simulink model "main_RI_LIEKF"  (R2023a)
settings: Solver=FixedStepAuto  StartTime=0.0  StopTime=220  FixedStep=0.01  RelTol=1e-3
InitFcn:
  | initNavigation0612_AOA;
values from neighbouring files (symbols this model uses):
  CF_enable = 0    [initNavigation.m]
  dt = 0.01    [initNavigation.m]
  dtDelay = -0.03    [initNavigation.m]
  g0 = 9.795    [initNavigation.m]
  gam0_rad = 0/57.3    (= 0)    [initNavigation.m]
  H_sensor_type = 0    [initNavigation.m]
  KF_enable = 1    [initNavigation.m]
  P0 = diag([1*ones(3,1);0.01*ones(3,1);0.1*ones(3,1);0.001*ones(3,1);0.00001*ones(3,1)])    [initNavigation.m]
  P0_RIEKF = diag([1*ones(3,1);0.01*ones(3,1);0.1*ones(3,1);0.001*ones(3,1);0.00001*ones(3,1);      0.01*ones(3,1);[0;2;2]/57.3;[0.1;0.1;0.1]])^2    [initNavigation.m]
  pd0 = 0    [initNavigation.m]
  pe0 = 0    [initNavigation.m]
  phi0_rad = 0/57.3    (= 0)    [initNavigation.m]
  pn0 = 0    [initNavigation.m]
  psi = -178    [initNavigation.m]
  psi0_rad = 0/57.3    (= 0)    [initNavigation.m]
  state_dim = 24    [initNavigation.m]
  Time = 0:0.01:(size(traindata.AttackAngle,1) - 1)*0.01    [NNLiftCoefficientFit.m]
  vd0 = 0    [initNavigation.m]
  ve0 = 0    [initNavigation.m]
  vn0 = 0    [initNavigation.m]
undefined symbols (not defined in the file or in its folder): DiscIntNeverNeededParam, Discrete, INS_CONST, INS_EXPORT, INS_PARAM, magnitude, p, param, pInitialization, sys
libraries: simulink x69, simulink_extras x64, dspstat3 x56, sharedtransform x49, ctrlSharedLib x36, sharedTrackingLibrary x17, FMT_Model_Lib x13, matrix_library x12, deeplib x4, dspsolvers x4, vrlib x4, aerolibconvert2 x1
(part 2 of 22)

== system main_RI_LIEKF/Sensor_Data_Process/Magn_Data_Process1/Mag_Data_Process ==
  mag_B_uT : Inport
  mag_valid : Inport  Port=2
  DCM_OB : Inport  Port=3
  GPS_Data : Inport  Port=4
  Bus Selector : BusSelector  OutputSignals=lat_gps,lon_gps
  Bus Selector1 : BusSelector  OutputSignals=fixtype_gps
  Compare To Constant : simulink/Logic and Bit Operations/Compare To Constant  relop=>=  const=1  OutDataTypeStr=boolean
  Mag_Quality_Estimate : Subsystem
  Scope : Scope
  WMM_Compensation : Subsystem
  WMM_LUT : Subsystem  mask{wmm_magnitude=INS_CONST.wmm_mag, wmm_declination=INS_CONST.wmm_dec, wmm_inclination=INS_CONST.wmm_inc, resolution=10}
      mask prompts: wmm_magnitude "WMM Magnitude Lookup Table"; wmm_declination "WMM Declination Lookup Table"; wmm_inclination "WMM Inclination Lookup Table"; resolution "Resolution (deg)"
  mag_normalized_B : Outport  VectorParamsAs1DForOutWhenUnconnected=off
  mag_quality : Outport  Port=2  VectorParamsAs1DForOutWhenUnconnected=off
  wires:
  Mag_Quality_Estimate/1(mag_quality) -> Scope/1, mag_quality/1
  WMM_LUT/3(inclination_deg) -> Mag_Quality_Estimate/2(nominal_inc_deg)
  mag_B_uT/1 -> WMM_Compensation/4(mag_B_uT)
  DCM_OB/1 -> WMM_Compensation/3(DCM_OB)
  WMM_Compensation/2(mag_normalized_O) -> Mag_Quality_Estimate/1(mag_normalized_O)
  WMM_LUT/1(magnitude_uT) -> WMM_Compensation/1(WMM_magnitude_uT)
  WMM_LUT/2(declination_deg) -> WMM_Compensation/2(WMM_declination_deg)
  GPS_Data/1 -> Bus Selector1/1, Bus Selector/1
  Bus Selector/1 -> WMM_LUT/1(lat_rad)  "<lat_gps>"
  Bus Selector/2 -> WMM_LUT/2(lon_rad)  "<lon_gps>"
  Compare To Constant/1 -> Mag_Quality_Estimate/3(pos_0_valid), WMM_Compensation/5(pos_0_valid)
  mag_valid/1 -> Mag_Quality_Estimate/4(mag_valid)
  WMM_Compensation/1(mag_normalized_B) -> mag_normalized_B/1
  Bus Selector1/1 -> Compare To Constant/1  "<fixtype_gps>"

== system main_RI_LIEKF/Sensor_Data_Process/Magn_Data_Process1/Sensor_Valid ==
  mag_B_gauss : Inport
  timestamp_ms : Inport  Port=2
  Compare To Constant4 : simulink/Logic and Bit Operations/Compare To Constant  relop=<  const=timeout  OutDataTypeStr=boolean
  Constant : Constant  Value=2  OutDataTypeStr=single
  Detect Change : simulink/Logic and Bit Operations/Detect Change  vinit=0  OutDataTypeStr=boolean
  Discrete-Time Integrator : DiscreteIntegrator  IntegratorMethod=Accumulation: Forward Euler  ExternalReset=sampled level  SampleTime=-1  OutDataTypeStr=uint32  SaturateOnIntegerOverflow=on  ICPrevOutput=DiscIntNeverNeededParam  ICPrevScaledInput=DiscIntNeverNeededParam
  Ever_Valid : Subsystem
  Interval Test1 : simulink/Logic and Bit Operations/Interval Test  IntervalClosedRight=off  uplimit=mag_max  IntervalClosedLeft=off  lowlimit=mag_min  OutDataTypeStr=boolean
  Logical Operator1 : Logic  Inputs=1  AllPortsSameDT=off  OutDataTypeStr=boolean
  Logical Operator4 : Logic  Inputs=3  AllPortsSameDT=off  OutDataTypeStr=boolean
  valid : Outport  VectorParamsAs1DForOutWhenUnconnected=off
  wires:
  Logical Operator4/1 -> valid/1
  Compare To Constant4/1 -> Logical Operator4/2
  Discrete-Time Integrator/1 -> Compare To Constant4/1
  Detect Change/1 -> Ever_Valid/1(in), Discrete-Time Integrator/2
  Constant/1 -> Discrete-Time Integrator/1
  Logical Operator1/1 -> Logical Operator4/1
  timestamp_ms/1 -> Detect Change/1
  mag_B_gauss/1 -> Interval Test1/1
  Interval Test1/1 -> Logical Operator1/1
  Ever_Valid/1(out) -> Logical Operator4/3

== system main_RI_LIEKF/Sensor_Data_Process/Subsystem/TD_baro ==
  H_baro : Inport
  Constant1 : Constant  Value=dt  OutDataTypeStr=single
  Constant3 : Constant  Value=0.1  OutDataTypeStr=single
  Constant4 : Constant  Value=900  OutDataTypeStr=single
  Delay1 : Delay  DelayLength=1  InitialConditionSource=Input port
      settings: InputPortMap=u0,p4
  MATLAB Function2 : MATLAB Function  TreatAsAtomicUnit=on
  Memory : Memory  InheritSampleTime=on
  Scope : Scope  NumInputPorts=3
  vH_baro_TD : Outport
  H_baro_TD : Outport  Port=2
  wires:
  MATLAB Function2/2(u2) -> Memory/1
  MATLAB Function2/1(u1) -> Delay1/1
  Constant4/1 -> MATLAB Function2/6(r)
  Constant1/1 -> MATLAB Function2/1(T)
  Constant3/1 -> MATLAB Function2/5(h)
  Memory/1 -> Scope/2, vH_baro_TD/1, MATLAB Function2/4("u2 ")
  H_baro/1 -> Scope/1, MATLAB Function2/2(u0), Delay1/2
  Delay1/1 -> MATLAB Function2/3("u1 "), Scope/3, H_baro_TD/1

== system main_RI_LIEKF/Sensor_Data_Process/TOF_Data_Process/TD_baro ==
  H_TOF : Inport
  Constant1 : Constant  Value=dt  OutDataTypeStr=single
  Constant3 : Constant  Value=0.04  OutDataTypeStr=single
  Constant4 : Constant  Value=600  OutDataTypeStr=single
  Delay1 : Delay  DelayLength=1  InitialConditionSource=Input port
      settings: InputPortMap=u0,p4
  MATLAB Function2 : MATLAB Function  TreatAsAtomicUnit=on
  Memory : Memory  InheritSampleTime=on
  Scope : Scope  NumInputPorts=3
  vH_TOF_TD : Outport
  H_TOF_TD : Outport  Port=2
  wires:
  MATLAB Function2/2(u2) -> Memory/1
  MATLAB Function2/1(u1) -> Delay1/1
  Constant4/1 -> MATLAB Function2/6(r)
  Constant1/1 -> MATLAB Function2/1(T)
  Constant3/1 -> MATLAB Function2/5(h)
  Memory/1 -> Scope/2, vH_TOF_TD/1, MATLAB Function2/4("u2 ")
  H_TOF/1 -> Scope/1, MATLAB Function2/2(u0), Delay1/2
  Delay1/1 -> MATLAB Function2/3("u1 "), Scope/3, H_TOF_TD/1

== system main_RI_LIEKF/Sensor_Data_Process/TOF_Data_Process/reinit_TOF ==
  QGC_sensor_reinit : Inport
  Data : Inport  Port=2
  Detect Increase : simulink/Logic and Bit Operations/Detect Increase  vinit=0.0  OutDataTypeStr=boolean
  Switch : Switch  Criteria=u2 > Threshold  SaturateOnIntegerOverflow=off  InputSameDT=off
  Unit Delay : UnitDelay  SampleTime=-1  HasFrameUpgradeWarning=on
  dataout : Outport
  wires:
  QGC_sensor_reinit/1 -> Detect Increase/1
  Detect Increase/1 -> Switch/2
  Switch/1 -> Unit Delay/1, dataout/1
  Data/1 -> Switch/1
  Unit Delay/1 -> Switch/3

== system main_RI_LIEKF/Sensor_Data_Process/baro_Data_Process/Pressure2Height ==
  baro : Inport
  Add : Sum  Inputs=+-
  Constant : Constant  OutDataTypeStr=single
  Constant1 : Constant  Value=1/5.255  OutDataTypeStr=single
  Gain : Gain  Gain=1/1.01325
  Gain1 : Gain  Gain=44330
  Math Function : Math  Operator=pow  SignedPower=on
  H_baro : Outport
  wires:
  baro/1 -> Gain/1
  Gain1/1 -> H_baro/1
  Add/1 -> Gain1/1
  Constant/1 -> Add/1
  Math Function/1 -> Add/2
  Constant1/1 -> Math Function/2
  Gain/1 -> Math Function/1

== system main_RI_LIEKF/Sensor_Data_Process/baro_Data_Process/TD_baro ==
  H_baro : Inport
  Constant1 : Constant  Value=dt  OutDataTypeStr=single
  Constant3 : Constant  Value=0.23  OutDataTypeStr=single
  Constant4 : Constant  Value=900  OutDataTypeStr=single
  Delay1 : Delay  DelayLength=1  InitialConditionSource=Input port
      settings: InputPortMap=u0,p4
  MATLAB Function2 : MATLAB Function  TreatAsAtomicUnit=on
  Memory : Memory  InheritSampleTime=on
  Scope : Scope  NumInputPorts=3
  vH_baro_TD : Outport
  H_baro_TD : Outport  Port=2
  wires:
  MATLAB Function2/2(u2) -> Memory/1
  MATLAB Function2/1(u1) -> Delay1/1
  Constant4/1 -> MATLAB Function2/6(r)
  Constant1/1 -> MATLAB Function2/1(T)
  Constant3/1 -> MATLAB Function2/5(h)
  Memory/1 -> Scope/2, vH_baro_TD/1, MATLAB Function2/4("u2 ")
  H_baro/1 -> Scope/1, MATLAB Function2/2(u0), Delay1/2
  Delay1/1 -> MATLAB Function2/3("u1 "), Scope/3, H_baro_TD/1

== system main_RI_LIEKF/Sensor_Data_Process/baro_Data_Process/TemCompensate1 ==
  baro_tem : Inport
  Add : Sum  Inputs=+++
  Constant2 : Constant  Value=-1663  OutDataTypeStr=single
  Gain : Gain  Gain=-1.6
  Gain1 : Gain  Gain=102.5
  Product : Product
  bias : Outport
  wires:
  baro_tem/1 -> Gain1/1, Product/2, Product/1
  Constant2/1 -> Add/3
  Product/1 -> Gain/1
  Gain/1 -> Add/1
  Add/1 -> bias/1
  Gain1/1 -> Add/2

== system main_RI_LIEKF/Sensor_Data_Process/baro_Data_Process/reinit_baro0 ==
  QGC_sensor_reinit : Inport
  Data : Inport  Port=2
  Detect Increase : simulink/Logic and Bit Operations/Detect Increase  vinit=0.0  OutDataTypeStr=boolean
  Switch : Switch  Criteria=u2 > Threshold  SaturateOnIntegerOverflow=off  InputSameDT=off
  Unit Delay : UnitDelay  SampleTime=-1  HasFrameUpgradeWarning=on
  dataout : Outport
  wires:
  QGC_sensor_reinit/1 -> Detect Increase/1
  Detect Increase/1 -> Switch/2
  Switch/1 -> Unit Delay/1, dataout/1
  Data/1 -> Switch/1
  Unit Delay/1 -> Switch/3

== system main_RI_LIEKF/Sensor_Data_Process/baro_Data_Process/reinit_baro1 ==
  QGC_sensor_reinit : Inport
  Data : Inport  Port=2
  Detect Increase : simulink/Logic and Bit Operations/Detect Increase  vinit=0.0  OutDataTypeStr=boolean
  Switch : Switch  Criteria=u2 > Threshold  SaturateOnIntegerOverflow=off  InputSameDT=off
  Unit Delay : UnitDelay  SampleTime=-1  HasFrameUpgradeWarning=on
  dataout : Outport
  wires:
  Unit Delay/1 -> Switch/3
  Data/1 -> Switch/1
  Switch/1 -> dataout/1, Unit Delay/1
  Detect Increase/1 -> Switch/2
  QGC_sensor_reinit/1 -> Detect Increase/1

== system main_RI_LIEKF/State estimation/0609bk/Bus_Constructor ==
  INSstate : Inport
  Bus Creator : BusCreator  Inputs=1
  Bus Creator2 : BusCreator  Inputs=6
  Bus Selector : BusSelector  OutputSignals=RotationData.DCM_b_n,INSstate_v,INSstste_p,bg,ba
  Demux : Demux  Outputs=3
  Demux1 : Demux  Outputs=3
  Scope : Scope  NumInputPorts=2
  TranslationData : Outport
  RotationData : Outport  Port=2
  wires:
  Bus Selector/5 -> Scope/2  "<ba>"
  Bus Selector/4 -> Scope/1  "<bg>"
  Bus Selector/3 -> Demux1/1  "<INSstste_p>"
  Bus Creator/1 -> RotationData/1
  Bus Selector/1 -> Bus Creator/1  "<DCM_b_n>"
  INSstate/1 -> Bus Selector/1
  Demux/2 -> Bus Creator2/2  "ve_m/s"
  Bus Creator2/1 -> TranslationData/1
  Demux/3 -> Bus Creator2/3  "vd_m/s"
  Demux1/2 -> Bus Creator2/5  "pe_m"
  Demux1/1 -> Bus Creator2/4  "pn_m"
  Demux1/3 -> Bus Creator2/6  "H_m"
  Bus Selector/2 -> Demux/1  "<INSstate_v>"
  Demux/1 -> Bus Creator2/1  "vn_m/s"

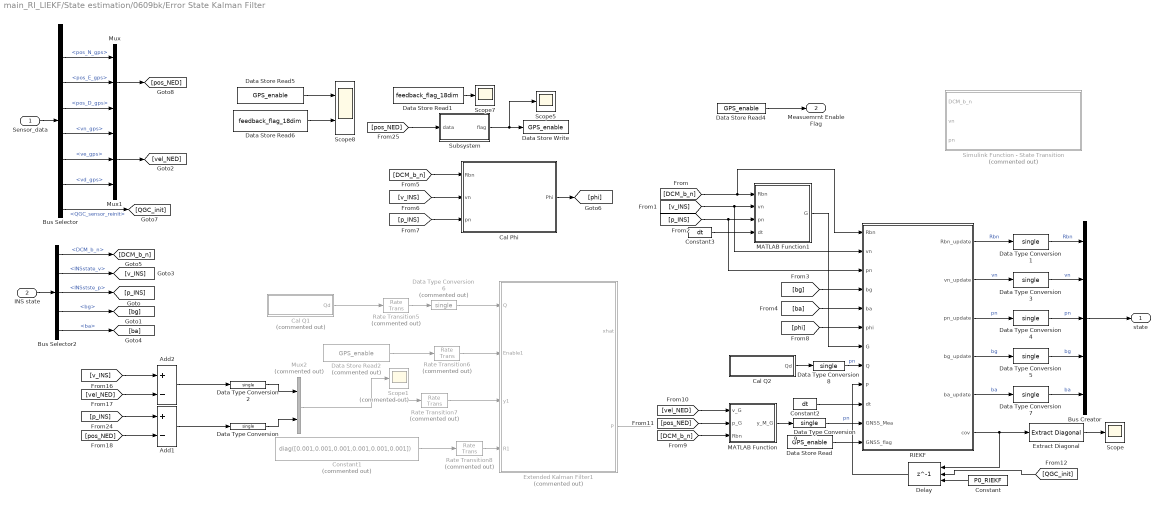
== system main_RI_LIEKF/State estimation/0609bk/Error State Kalman Filter ==
  Sensor_data : Inport
  INS state : Inport  Port=2
  Add1 : Sum  Inputs=+-
  Add2 : Sum  Inputs=+-
  Bus Creator : BusCreator  Inputs=5
  Bus Selector : BusSelector  OutputSignals=QGC_sensor_reinit,GPS_Data.pos_N_gps,GPS_Data.pos_E_gps,GPS_Data.pos_D_gps,GPS_Data.vn_gps,GPS_Data.ve_gps,GPS_Data.vd_gps,QGC_sensor_reinit
  Bus Selector2 : BusSelector  OutputSignals=RotationData.DCM_b_n,INSstate_v,INSstste_p,bg,ba
  Cal Phi : Subsystem
  Cal Q1 : Subsystem  Commented=on
  Cal Q2 : Subsystem
  Constant : Constant  Value=P0_RIEKF
  Constant1 : Constant  Commented=on  Value=diag([0.001,0.001,0.001,0.001,0.001,0.001])  OutDataTypeStr=single
  Constant2 : Constant  Value=dt  OutDataTypeStr=single
  Constant3 : Constant  Value=dt  OutDataTypeStr=single
  Data Store Read : DataStoreRead  DataStoreName=GPS_enable  IndexOptions=Index vector (dialog)  Indices=1  OutputSizes=1
  Data Store Read1 : DataStoreRead  DataStoreName=feedback_flag_18dim  IndexOptions=Index vector (dialog)  Indices=1  OutputSizes=1
  Data Store Read2 : DataStoreRead  Commented=on  DataStoreName=GPS_enable  IndexOptions=Index vector (dialog)  Indices=1  OutputSizes=1
  Data Store Read4 : DataStoreRead  DataStoreName=GPS_enable  IndexOptions=Index vector (dialog)  Indices=1  OutputSizes=1
  Data Store Read5 : DataStoreRead  DataStoreName=GPS_enable  IndexOptions=Index vector (dialog)  Indices=1  OutputSizes=1
  Data Store Read6 : DataStoreRead  DataStoreName=feedback_flag_18dim  IndexOptions=Index vector (dialog)  Indices=1  OutputSizes=1
  Data Store Write : DataStoreWrite  DataStoreName=GPS_enable  IndexOptions=Index vector (dialog)  Indices=1  OutputSizes=1
  Data Type Conversion{,1..5,7..9} (9 alike) : DataTypeConversion  OutDataTypeStr=single  SaturateOnIntegerOverflow=off  RndMeth=Floor
  Data Type Conversion6 : DataTypeConversion  Commented=on  OutDataTypeStr=single  SaturateOnIntegerOverflow=off  RndMeth=Floor
  Delay : Delay  DelayLength=1  InitialConditionSource=Input port  ExternalReset=Level hold
      settings: InputPortMap=u0,r5,p4
  Extended Kalman Filter1 : Subsystem  Commented=on  mask(Extended Kalman Filter){StateTransitionFcn=stateTransitionFcn_Dyn, HasStateTransitionJacobianFcn=off, StateTransitionJacobianFcn=stateTransitionJacobianFcn_Dyn, HasAdditiveProcessNoise=Nonadditive, ProcessNoise=1, HasTimeVaryingProcessNoise=on, HasStateTransitionFcnExtraArgument=0, InitialState=zeros(15,1), InitialStateCovariance=P0_RIEKF, MeasurementFcn1=GPSMeasurementFcn_Dyn, HasMeasurementJacobianFcn1=off, MeasurementJacobianFcn1=, HasMeasurementEnablePort1=on, HasAdditiveMeasurementNoise1=Nonadditive, MeasurementNoise1=1, HasTimeVaryingMeasurementNoise1=on, HasMeasurementFcnExtraArgument1=0, HasMeasurementWrapping1=off, MeasurementFcn2=ZUPTMeasurementFcn2, HasMeasurementJacobianFcn2=off, MeasurementJacobianFcn2=, HasMeasurementEnablePort2=on, HasAdditiveMeasurementNoise2=Nonadditive, MeasurementNoise2=1, HasTimeVaryingMeasurementNoise2=on, HasMeasurementFcnExtraArgument2=0, HasMeasurementWrapping2=off, MeasurementFcn3=ZUPTMeasurementFcn2, HasMeasurementJacobianFcn3=off, MeasurementJacobianFcn3=, HasMeasurementEnablePort3=on, HasAdditiveMeasurementNoise3=Nonadditive, MeasurementNoise3=1, HasTimeVaryingMeasurementNoise3=on, HasMeasurementFcnExtraArgument3=0, HasMeasurementWrapping3=off, MeasurementFcn4=myMeasurementFcn, HasMeasurementJacobianFcn4=off, MeasurementJacobianFcn4=, HasMeasurementEnablePort4=off, HasAdditiveMeasurementNoise4=Additive, MeasurementNoise4=1, HasTimeVaryingMeasurementNoise4=off, HasMeasurementFcnExtraArgument4=0, HasMeasurementWrapping4=off, MeasurementFcn5=myMeasurementFcn, HasMeasurementJacobianFcn5=off, MeasurementJacobianFcn5=, HasMeasurementEnablePort5=off, HasAdditiveMeasurementNoise5=Additive, MeasurementNoise5=1, HasTimeVaryingMeasurementNoise5=off, HasMeasurementFcnExtraArgument5=0, HasMeasurementWrapping5=off, EnableMultirate=off, StateTransitionFcnSampleTime=0.01, MeasurementFcn1SampleTime=0.2, MeasurementFcn2SampleTime=0.01, MeasurementFcn3SampleTime=1, MeasurementFcn4SampleTime=1, MeasurementFcn5SampleTime=1, UseCurrentEstimator=on, OutputStateCovariance=on, DataType=single, SampleTime=0.01, NumberOfMeasurements=1}
      mask prompts: HasStateTransitionJacobianFcn "shared_tracking:blocks:maskPromptEKFJacobian"; HasTimeVaryingProcessNoise "shared_tracking:blocks:maskPromptEKFUKFTimeVarying"; HasMeasurementJacobianFcn1 "shared_tracking:blocks:maskPromptEKFJacobian"; HasMeasurementEnablePort1 "shared_tracking:blocks:maskPromptEnablePort"; HasTimeVaryingMeasurementNoise1 "shared_tracking:blocks:maskPromptEKFUKFTimeVarying"; HasMeasurementWrapping1 "shared_tracking:blocks:maskPromptEKFUKFMeasurementWrapping"; HasMeasurementJacobianFcn2 "shared_tracking:blocks:maskPromptEKFJacobian"; HasMeasurementEnablePort2 "shared_tracking:blocks:maskPromptEnablePort"; HasTimeVaryingMeasurementNoise2 "shared_tracking:blocks:maskPromptEKFUKFTimeVarying"; HasMeasurementWrapping2 "shared_tracking:blocks:maskPromptEKFUKFMeasurementWrapping"; HasMeasurementJacobianFcn3 "shared_tracking:blocks:maskPromptEKFJacobian"; HasMeasurementEnablePort3 "shared_tracking:blocks:maskPromptEnablePort"; HasTimeVaryingMeasurementNoise3 "shared_tracking:blocks:maskPromptEKFUKFTimeVarying"; HasMeasurementWrapping3 "shared_tracking:blocks:maskPromptEKFUKFMeasurementWrapping"; HasMeasurementJacobianFcn4 "shared_tracking:blocks:maskPromptEKFJacobian"; HasMeasurementEnablePort4 "shared_tracking:blocks:maskPromptEnablePort"; HasTimeVaryingMeasurementNoise4 "shared_tracking:blocks:maskPromptEKFUKFTimeVarying"; HasMeasurementWrapping4 "shared_tracking:blocks:maskPromptEKFUKFMeasurementWrapping"; HasMeasurementJacobianFcn5 "shared_tracking:blocks:maskPromptEKFJacobian"; HasMeasurementEnablePort5 "shared_tracking:blocks:maskPromptEnablePort"; HasTimeVaryingMeasurementNoise5 "shared_tracking:blocks:maskPromptEKFUKFTimeVarying"; HasMeasurementWrapping5 "shared_tracking:blocks:maskPromptEKFUKFMeasurementWrapping"; EnableMultirate "shared_tracking:blocks:maskPromptEnableMultirate"; StateTransitionFcnSampleTime "shared_tracking:blocks:maskPromptStateTransition"; MeasurementFcn1SampleTime "shared_tracking:blocks:maskPromptMeasurement1"; MeasurementFcn2SampleTime "shared_tracking:blocks:maskPromptMeasurement2"; MeasurementFcn3SampleTime "shared_tracking:blocks:maskPromptMeasurement3"; MeasurementFcn4SampleTime "shared_tracking:blocks:maskPromptMeasurement4"; MeasurementFcn5SampleTime "shared_tracking:blocks:maskPromptMeasurement5"; UseCurrentEstimator "shared_tracking:blocks:maskPromptUseCurrentEstimator"; OutputStateCovariance "shared_tracking:blocks:maskPromptOutputStateCovariance"; DataType "shared_tracking:blocks:maskPromptDataType"; SampleTime "shared_tracking:blocks:maskPromptSampleTime"
      mask help: shared_tracking:blocks:maskPromptEKFDescription
      mask init:
      | matlabshared.tracking.internal.blocks.maskInitializationScriptEKF
      mask Help: eval('matlabshared.tracking.internal.blocks.controlIdentLaunchDocPage(''EKF'')')
      mask Callback HasStateTransitionJacobianFcn: matlabshared.tracking.internal.blocks.dialogCallbacksEKFUKFPF(gcbh(),'checkBoxHasJacobianFcn','StateTransition');
      mask TypeOptions HasAdditiveProcessNoise: shared_tracking:blocks:maskPromptEKFUKFAdditiveNoise | shared_tracking:blocks:maskPromptEKFUKFNonAdditiveNoise
      mask Callback HasTimeVaryingProcessNoise: matlabshared.tracking.internal.blocks.dialogCallbacksEKFUKFPF(gcbh,'checkboxIsCovarianceTimeVarying','HasTimeVaryingProcessNoise','ProcessNoise')
      mask Callback HasMeasurementJacobianFcn1: matlabshared.tracking.internal.blocks.dialogCallbacksEKFUKFPF(gcbh(),'checkBoxHasJacobianFcn','Measurement','1');
      mask TypeOptions HasAdditiveMeasurementNoise1: shared_tracking:blocks:maskPromptEKFUKFAdditiveNoise | shared_tracking:blocks:maskPromptEKFUKFNonAdditiveNoise
      mask Callback HasTimeVaryingMeasurementNoise1: matlabshared.tracking.internal.blocks.dialogCallbacksEKFUKFPF(gcbh,'checkboxIsCovarianceTimeVarying','HasTimeVaryingMeasurementNoise1','MeasurementNoise1')
      mask Callback HasMeasurementJacobianFcn2: matlabshared.tracking.internal.blocks.dialogCallbacksEKFUKFPF(gcbh(),'checkBoxHasJacobianFcn','Measurement','2');
      mask TypeOptions HasAdditiveMeasurementNoise2: shared_tracking:blocks:maskPromptEKFUKFAdditiveNoise | shared_tracking:blocks:maskPromptEKFUKFNonAdditiveNoise
      mask Callback HasTimeVaryingMeasurementNoise2: matlabshared.tracking.internal.blocks.dialogCallbacksEKFUKFPF(gcbh,'checkboxIsCovarianceTimeVarying','HasTimeVaryingMeasurementNoise2','MeasurementNoise2')
      mask Callback HasMeasurementJacobianFcn3: matlabshared.tracking.internal.blocks.dialogCallbacksEKFUKFPF(gcbh(),'checkBoxHasJacobianFcn','Measurement','3');
      mask TypeOptions HasAdditiveMeasurementNoise3: shared_tracking:blocks:maskPromptEKFUKFAdditiveNoise | shared_tracking:blocks:maskPromptEKFUKFNonAdditiveNoise
      mask Callback HasTimeVaryingMeasurementNoise3: matlabshared.tracking.internal.blocks.dialogCallbacksEKFUKFPF(gcbh,'checkboxIsCovarianceTimeVarying','HasTimeVaryingMeasurementNoise3','MeasurementNoise3')
      mask Callback HasMeasurementJacobianFcn4: matlabshared.tracking.internal.blocks.dialogCallbacksEKFUKFPF(gcbh(),'checkBoxHasJacobianFcn','Measurement','4');
      mask TypeOptions HasAdditiveMeasurementNoise4: shared_tracking:blocks:maskPromptEKFUKFAdditiveNoise | shared_tracking:blocks:maskPromptEKFUKFNonAdditiveNoise
      mask Callback HasTimeVaryingMeasurementNoise4: matlabshared.tracking.internal.blocks.dialogCallbacksEKFUKFPF(gcbh,'checkboxIsCovarianceTimeVarying','HasTimeVaryingMeasurementNoise4','MeasurementNoise4')
      mask Callback HasMeasurementJacobianFcn5: matlabshared.tracking.internal.blocks.dialogCallbacksEKFUKFPF(gcbh(),'checkBoxHasJacobianFcn','Measurement','5');
      mask TypeOptions HasAdditiveMeasurementNoise5: shared_tracking:blocks:maskPromptEKFUKFAdditiveNoise | shared_tracking:blocks:maskPromptEKFUKFNonAdditiveNoise
      mask Callback HasTimeVaryingMeasurementNoise5: matlabshared.tracking.internal.blocks.dialogCallbacksEKFUKFPF(gcbh,'checkboxIsCovarianceTimeVarying','HasTimeVaryingMeasurementNoise5','MeasurementNoise5')
      mask Callback EnableMultirate: matlabshared.tracking.internal.blocks.dialogCallbacksEKFUKFPF(gcbh,'checkBoxHasMultirate')
      mask TypeOptions DataType: shared_tracking:blocks:maskPromptDouble | shared_tracking:blocks:maskPromptSingle
      mask Callback NumberOfMeasurements: matlabshared.tracking.internal.blocks.dialogCallbacksEKFUKFPF(gcbh,'editboxNumberOfMeasurements','MeasurementFcn');
      mask DialogControl DescGroupVar Prompt: shared_tracking:blocks:maskPromptEKFTitle
      mask DialogControl TabSystemModel Prompt: shared_tracking:blocks:maskPromptSystemModel
      mask DialogControl GroupStateTransition Prompt: shared_tracking:blocks:maskPromptStateTransition
      mask DialogControl StateTransitionFunctionText Prompt: shared_tracking:blocks:maskPromptFunction
      mask DialogControl HasStateTransitionJacobianFcn Prompt: Jacobian
      mask DialogControl ProcessNoiseText Prompt: shared_tracking:blocks:maskPromptEKFUKFProcessNoise
      mask DialogControl ProcessNoiseCovarianceText Prompt: shared_tracking:blocks:maskPromptCovariance
      mask DialogControl HasTimeVaryingProcessNoise Prompt: Time-varying
      mask DialogControl InitializationContainer Prompt: shared_tracking:blocks:maskPromptInitialization
      mask DialogControl InitialStateText Prompt: shared_tracking:blocks:maskPromptEKFUKFInitialState
      mask DialogControl InitialCovarianceText Prompt: shared_tracking:blocks:maskPromptEKFUKFInitialCovariance
      mask DialogControl GroupMeasurement1 Prompt: shared_tracking:blocks:maskPromptMeasurement1
      mask DialogControl MeasurementFunction1Text Prompt: shared_tracking:blocks:maskPromptFunction
      mask DialogControl HasMeasurementJacobianFcn1 Prompt: Jacobian
      mask DialogControl HasMeasurementEnablePort1 Prompt: Add Enable port
      mask DialogControl MeasurementNoiseText1 Prompt: shared_tracking:blocks:maskPromptEKFUKFMeasurementNoise
      mask DialogControl MeasurementNoiseCovarianceText1 Prompt: shared_tracking:blocks:maskPromptCovariance
      mask DialogControl HasTimeVaryingMeasurementNoise1 Prompt: Time-varying
      mask DialogControl HasMeasurementWrapping1 Prompt: Has measurement wrapping
      mask DialogControl GroupMeasurement2 Prompt: shared_tracking:blocks:maskPromptMeasurement2
      mask DialogControl MeasurementFunction2Text Prompt: shared_tracking:blocks:maskPromptFunction
      mask DialogControl HasMeasurementJacobianFcn2 Prompt: Jacobian
      mask DialogControl HasMeasurementEnablePort2 Prompt: Add Enable port
      mask DialogControl MeasurementNoiseText2 Prompt: shared_tracking:blocks:maskPromptEKFUKFMeasurementNoise
      mask DialogControl MeasurementNoiseCovarianceText2 Prompt: shared_tracking:blocks:maskPromptCovariance
      mask DialogControl HasTimeVaryingMeasurementNoise2 Prompt: Time-varying
      mask DialogControl HasMeasurementWrapping2 Prompt: Has measurement wrapping
      mask DialogControl GroupMeasurement3 Prompt: shared_tracking:blocks:maskPromptMeasurement3
      mask DialogControl MeasurementFunction3Text Prompt: shared_tracking:blocks:maskPromptFunction
      mask DialogControl HasMeasurementJacobianFcn3 Prompt: Jacobian
      mask DialogControl HasMeasurementEnablePort3 Prompt: Add Enable port
      mask DialogControl MeasurementNoiseText3 Prompt: shared_tracking:blocks:maskPromptEKFUKFMeasurementNoise
      mask DialogControl MeasurementNoiseCovarianceText3 Prompt: shared_tracking:blocks:maskPromptCovariance
      mask DialogControl HasTimeVaryingMeasurementNoise3 Prompt: Time-varying
      mask DialogControl HasMeasurementWrapping3 Prompt: Has measurement wrapping
      mask DialogControl GroupMeasurement4 Prompt: shared_tracking:blocks:maskPromptMeasurement4
      mask DialogControl MeasurementFunction4Text Prompt: shared_tracking:blocks:maskPromptFunction
      mask DialogControl HasMeasurementJacobianFcn4 Prompt: Jacobian
      mask DialogControl HasMeasurementEnablePort4 Prompt: Add Enable port
      mask DialogControl MeasurementNoiseText4 Prompt: shared_tracking:blocks:maskPromptEKFUKFMeasurementNoise
      mask DialogControl MeasurementNoiseCovarianceText4 Prompt: shared_tracking:blocks:maskPromptCovariance
      mask DialogControl HasTimeVaryingMeasurementNoise4 Prompt: Time-varying
      mask DialogControl HasMeasurementWrapping4 Prompt: Has measurement wrapping
      mask DialogControl GroupMeasurement5 Prompt: shared_tracking:blocks:maskPromptMeasurement5
      mask DialogControl MeasurementFunction5Text Prompt: shared_tracking:blocks:maskPromptFunction
      mask DialogControl HasMeasurementJacobianFcn5 Prompt: Jacobian
      mask DialogControl HasMeasurementEnablePort5 Prompt: Add Enable port
      mask DialogControl MeasurementNoiseText5 Prompt: shared_tracking:blocks:maskPromptEKFUKFMeasurementNoise
      mask DialogControl MeasurementNoiseCovarianceText5 Prompt: shared_tracking:blocks:maskPromptCovariance
      mask DialogControl HasTimeVaryingMeasurementNoise5 Prompt: Time-varying
      mask DialogControl HasMeasurementWrapping5 Prompt: Has measurement wrapping
      mask DialogControl AddMeasurement Prompt: shared_tracking:blocks:maskPromptAddMeasurement
      mask DialogControl AddMeasurement Callback: matlabshared.tracking.internal.blocks.dialogCallbacksEKFUKFPF(gcbh,'buttonAddMeasurement','MeasurementFcn');
      mask DialogControl RemoveMeasurement Prompt: shared_tracking:blocks:maskPromptRemoveMeasurement
      mask DialogControl RemoveMeasurement Callback: matlabshared.tracking.internal.blocks.dialogCallbacksEKFUKFPF(gcbh,'buttonRemoveMeasurement','MeasurementFcn');
      mask DialogControl TabMultirate Prompt: shared_tracking:blocks:maskPromptEKFUKFMultirate
      mask DialogControl GroupMultirate Prompt: shared_tracking:blocks:maskPromptEKFUKFMultirate
      mask DialogControl EnableMultirate Prompt: Enable multirate operation
      mask DialogControl GroupMultirateSampleTimes Prompt: shared_tracking:blocks:maskPromptSampleTimeNoInheritance
      mask DialogControl StateTransitionFcnSampleTime Prompt: State Transition
      mask DialogControl MeasurementFcn1SampleTime Prompt: Measurement 1
      mask DialogControl MeasurementFcn2SampleTime Prompt: Measurement 2
      mask DialogControl MeasurementFcn3SampleTime Prompt: Measurement 3
      mask DialogControl MeasurementFcn4SampleTime Prompt: Measurement 4
      mask DialogControl MeasurementFcn5SampleTime Prompt: Measurement 5
      mask DialogControl ContainerSettings Prompt: shared_tracking:blocks:maskPromptEKFUKFSettings
      mask DialogControl UseCurrentEstimator Prompt: Use the current measurements to improve state estimates
      mask DialogControl OutputStateCovariance Prompt: Output state estimation error covariance
      mask DialogControl DataType Prompt: Data type:
      mask DialogControl SampleTime Prompt: Sample time:
  Extract Diagonal : matrix_library/Extract Diagonal
      settings: LibrarySourceBlock=|
      | simulink/Matrix
      | Operations/Extract Diagonal
  MATLAB Function : MATLAB Function  TreatAsAtomicUnit=on
  MATLAB Function1 : MATLAB Function  TreatAsAtomicUnit=on
  Mux : Mux  Inputs=3
  Mux1 : Mux  Inputs=3
  Mux2 : Mux  Commented=on  Inputs=2
  RIEKF : MATLAB Function  TreatAsAtomicUnit=on
  Rate Transition{5..8} (4 alike) : RateTransition  Commented=on  OutPortSampleTime=dt
  Scope : Scope
  Scope1 : Scope  Commented=on
  Scope5 : Scope
  Scope7 : Scope
  Scope8 : Scope  NumInputPorts=2
  Simulink Function - State Transition : Subsystem  Commented=on  TreatAsAtomicUnit=on
  Subsystem : Subsystem
  state : Outport
  Measuemrnt Enable Flag : Outport  Port=2
  wires:
  [QGC_init] -> Delay/2
  Bus Selector/8 -> [QGC_init]  "<QGC_sensor_reinit>"
  Bus Selector2/3 -> [p_INS]  "<INSstste_p>"
  Bus Selector2/1 -> [DCM_b_n]  "<DCM_b_n>"
  Bus Selector2/5 -> [ba]  "<ba>"
  Bus Selector2/4 -> [bg]  "<bg>"
  INS state/1 -> Bus Selector2/1
  Bus Selector/4 -> Mux/3  "<pos_D_gps>"
  Bus Selector/2 -> Mux/1  "<pos_N_gps>"
  Bus Selector/3 -> Mux/2  "<pos_E_gps>"
  Bus Selector/7 -> Mux1/3  "<vd_gps>"
  Bus Selector/5 -> Mux1/1  "<vn_gps>"
  Mux1/1 -> [vel_NED]
  Sensor_data/1 -> Bus Selector/1
  Bus Selector/6 -> Mux1/2  "<ve_gps>"
  Data Store Read1/1 -> Scope7/1
  [pos_NED] -> Subsystem/1(data)
  Subsystem/1(flag) -> Data Store Write/1, Scope5/1
  Constant1/1 -> Rate Transition8/1
  Extended Kalman Filter1/2(P) -> ?
  Rate Transition6/1 -> Extended Kalman Filter1/2(Enable1)
  Rate Transition7/1 -> Extended Kalman Filter1/3(y1)
  Rate Transition8/1 -> Extended Kalman Filter1/4(R1)
  Cal Q1/1(Qd) -> Rate Transition5/1
  Rate Transition5/1 -> Data Type Conversion6/1
  Data Type Conversion6/1 -> Extended Kalman Filter1/1(Q)
  Data Store Read5/1 -> Scope8/1
  Data Store Read6/1 -> Scope8/2
  Bus Selector2/2 -> [v_INS]  "<INSstate_v>"
  Mux/1 -> [pos_NED]
  Data Store Read2/1 -> Rate Transition6/1
  Data Store Read4/1 -> Measuemrnt Enable Flag/1
  [vel_NED] -> Add2/2
  [pos_NED] -> Add1/2
  Data Type Conversion/1 -> Mux2/2
  Data Type Conversion2/1 -> Mux2/1
  Mux2/1 -> Scope1/1, Rate Transition7/1
  [v_INS] -> Add2/1
  [p_INS] -> Add1/1
  Add2/1 -> Data Type Conversion2/1
  Add1/1 -> Data Type Conversion/1
  [DCM_b_n] -> MATLAB Function1/1(Rbn), RIEKF/1(Rbn)
  [v_INS] -> RIEKF/2(vn), MATLAB Function1/2(vn)
  [p_INS] -> RIEKF/3(pn), MATLAB Function1/3(pn)
  RIEKF/1(Rbn_update) -> Data Type Conversion1/1  "Rbn"
  RIEKF/2(vn_update) -> Data Type Conversion3/1  "vn"
  RIEKF/3(pn_update) -> Data Type Conversion4/1  "pn"
  RIEKF/4(bg_update) -> Data Type Conversion5/1  "bg"
  RIEKF/5(ba_update) -> Data Type Conversion7/1  "ba"
  Bus Creator/1 -> state/1
  RIEKF/6(cov) -> Extract Diagonal/1, Delay/1
  Extract Diagonal/1 -> Scope/1
  Cal Q2/1(Qd) -> Data Type Conversion8/1
  [bg] -> RIEKF/4(bg)
  [ba] -> RIEKF/5(ba)
  [DCM_b_n] -> Cal Phi/1(Rbn)
  [v_INS] -> Cal Phi/2(vn)
  [p_INS] -> Cal Phi/3(pn)
  Cal Phi/1(Phi) -> [phi]
  [phi] -> RIEKF/6(phi)
  Delay/1 -> RIEKF/9(P)
  Constant/1 -> Delay/3
  MATLAB Function/1(y_M_G) -> Data Type Conversion9/1
  Data Store Read/1 -> RIEKF/12(GNSS_flag)
  [DCM_b_n] -> MATLAB Function/3(Rbn)
  [vel_NED] -> MATLAB Function/1(v_G)
  [pos_NED] -> MATLAB Function/2(p_G)
  Constant2/1 -> RIEKF/10(dt)
  Data Type Conversion1/1 -> Bus Creator/1  "Rbn"
  Data Type Conversion3/1 -> Bus Creator/2  "vn"
  Data Type Conversion4/1 -> Bus Creator/3  "pn"
  Data Type Conversion5/1 -> Bus Creator/4  "bg"
  Data Type Conversion7/1 -> Bus Creator/5  "ba"
  Data Type Conversion8/1 -> RIEKF/8(Q)  "pn"
  Data Type Conversion9/1 -> RIEKF/11(GNSS_Mea)  "pn"
  MATLAB Function1/1(G) -> RIEKF/7(G)
  Constant3/1 -> MATLAB Function1/4(dt)

== system main_RI_LIEKF/State estimation/0609bk/INS propogation ==
  note: q(1:3)
  Sensor_data : Inport
  state : Inport  Port=2
  Add : Sum  Inputs=+-
  Add1 : Sum  Inputs=+-
  Bus Creator : BusCreator  Inputs=7
  Bus Selector : BusSelector  OutputSignals=IMU_Data.gyro_B_rad/s_LPF,IMU_Data.accl_B_m/s2_LPF,MAGN_Data,QGC_sensor_reinit,GPS_Data.pos_N_gps,GPS_Data.pos_E_gps,GPS_Data.pos_D_gps,GPS_Data.vn_gps,GPS_Data.ve_gps,GPS_Data.vd_gps
  Bus Selector1 : BusSelector  OutputSignals=DCM_b_n
  Bus Selector2 : BusSelector  OutputSignals=Rbn,vn,pn,bg,ba
  Data Type Conversion : DataTypeConversion  OutDataTypeStr=single  SaturateOnIntegerOverflow=off  RndMeth=Floor
  Init_PVQ : Subsystem
  Memory2 : Memory
  Memory3 : Memory
  Mux : Mux  Inputs=3
  Mux1 : Mux  Inputs=3
  Zero : Constant  Value=zeros(3,1)  OutDataTypeStr=single
  att_update : Subsystem
  vel_pos_update : Subsystem
  INSstate : Outport
  wires:
  Bus Selector/2 -> [accl_raw]  "<accl_B_m/s2_LPF>"
  Bus Creator/1 -> INSstate/1
  att_update/1(att_update1) -> Bus Selector1/1, Bus Creator/1  "RotationData"
  vel_pos_update/1(p_k) -> Bus Creator/2  "INSstste_p"
  [QGC_init] -> Init_PVQ/1(QGC_sensor_reinit)
  vel_pos_update/2(V) -> Bus Creator/3  "INSstate_v"
  Bus Selector1/1 -> vel_pos_update/1(<DCM_b_n>)  "<DCM_b_n>"
  Bus Selector/1 -> [gyro_raw]  "<gyro_B_rad/s_LPF>"
  Bus Selector/4 -> [QGC_init]  "<QGC_sensor_reinit>"
  [Magn] -> Init_PVQ/3(Magn_B_guess_LPF)
  Data Type Conversion/1 -> Init_PVQ/5(vel_NED)
  [pos_NED] -> Init_PVQ/4(pos_NED)
  [QGC_init] -> vel_pos_update/5(QGC_init)
  Bus Selector/9 -> Mux1/2  "<ve_gps>"
  Init_PVQ/3(p0) -> vel_pos_update/4(p0)
  Init_PVQ/2(v0) -> vel_pos_update/3(v0)
  [accl_raw] -> Init_PVQ/2(accl_B_m/s2_LPF)
  Sensor_data/1 -> Bus Selector/1
  Mux1/1 -> [vel_NED]
  Bus Selector/3 -> [Magn]  "<MAGN_Data>"
  Bus Selector/6 -> Mux/2  "<pos_E_gps>"
  Add/1 -> Bus Creator/4, att_update/2(gyro)  "gyro_unbias"
  Bus Selector/5 -> Mux/1  "<pos_N_gps>"
  Bus Selector/8 -> Mux1/1  "<vn_gps>"
  Bus Selector/7 -> Mux/3  "<pos_D_gps>"
  [vel_NED] -> Data Type Conversion/1
  Bus Selector/10 -> Mux1/3  "<vd_gps>"
  [QGC_init] -> att_update/4(init_flag)
  Add1/1 -> Bus Creator/5, vel_pos_update/2(Ab)  "accl_unbias"
  Init_PVQ/1(quat_0) -> att_update/3(quat_0)
  Mux/1 -> [pos_NED]
  state/1 -> Bus Selector2/1
  Bus Selector2/1 -> [Rbn]  "<Rbn>"
  Bus Selector2/2 -> [vn]  "<vn>"
  Bus Selector2/3 -> [pn]  "<pn>"
  Bus Selector2/4 -> Memory2/1  "<bg>"
  Bus Selector2/5 -> Memory3/1  "<ba>"
  [gyro_raw] -> Add/1
  [Rbn] -> att_update/1(Rbn)
  [accl_raw] -> Add1/1
  [vn] -> vel_pos_update/7(vn)
  [pn] -> vel_pos_update/6(pn)
  [bg] -> Bus Creator/6  "bg"
  [ba] -> Bus Creator/7  "ba"
  Memory2/1 -> [bg]
  Memory3/1 -> [ba]
  [bg] -> ?
  [ba] -> ?
  Zero/1 -> Add/2, Add1/2

== system main_RI_LIEKF/State estimation/15dim KF1/Bus_Constructor ==
  INSstate : Inport
  Bus Creator : BusCreator  Inputs=2
  Bus Creator2 : BusCreator  Inputs=6
  Bus Selector : BusSelector  OutputSignals=RotationData.q_update,RotationData.DCM_b_n,INSstate_v,INSstste_p,INSstate_dg,INSstate_da
  Demux : Demux  Outputs=3
  Demux1 : Demux  Outputs=3
  Scope : Scope  NumInputPorts=2
  TranslationData : Outport
  RotationData : Outport  Port=2
  wires:
  Bus Selector/6 -> Scope/2  "<INSstate_da>"
  Bus Selector/5 -> Scope/1  "<INSstate_dg>"
  Bus Selector/4 -> Demux1/1  "<INSstste_p>"
  Bus Creator/1 -> RotationData/1
  Bus Selector/1 -> Bus Creator/1  "<q_update>"
  Bus Selector/2 -> Bus Creator/2  "<DCM_b_n>"
  INSstate/1 -> Bus Selector/1
  Demux/2 -> Bus Creator2/2  "ve_m/s"
  Bus Creator2/1 -> TranslationData/1
  Demux/3 -> Bus Creator2/3  "vd_m/s"
  Demux1/2 -> Bus Creator2/5  "pe_m"
  Demux1/1 -> Bus Creator2/4  "pn_m"
  Demux1/3 -> Bus Creator2/6  "H_m"
  Bus Selector/3 -> Demux/1  "<INSstate_v>"
  Demux/1 -> Bus Creator2/1  "vn_m/s"

== system main_RI_LIEKF/State estimation/15dim KF1/Error State Kalman Filter ==
  Sensor_data : Inport
  INS state : Inport  Port=2
  Add : Sum  Inputs=+-
  Bus Creator : BusCreator  Inputs=5
  Bus Selector : BusSelector  OutputSignals=QGC_sensor_reinit,GPS_Data.pos_N_gps,GPS_Data.pos_E_gps,GPS_Data.pos_D_gps,GPS_Data.vn_gps,GPS_Data.ve_gps,GPS_Data.vd_gps,vicon.vicon_posxyz,QGC_sensor_reinit
  Bus Selector2 : BusSelector  OutputSignals=RotationData.DCM_b_n,INSstate_v,INSstste_p,INSstate_w,INSstate_fb
  Cal Phi : Subsystem
  Cal Q : Subsystem
  Constant6 : Constant  Value=[eye(3),zeros(3,12)]  OutDataTypeStr=single
  Constant7 : Constant  Value=zeros(15,1)  OutDataTypeStr=single
  Data Store Read1 : DataStoreRead  DataStoreName=feedback_flag  IndexOptions=Index vector (dialog)  Indices=1  OutputSizes=1
  Data Store Read2 : DataStoreRead  DataStoreName=feedback_flag  IndexOptions=Index vector (dialog)  Indices=1  OutputSizes=1
  Data Type Conversion{1..3,5} (4 alike) : DataTypeConversion  OutDataTypeStr=single  SaturateOnIntegerOverflow=off  RndMeth=Floor
  Extract Diagonal : matrix_library/Extract Diagonal
  GNSS/INS Kalman Filter1 : Subsystem  AncestorBlock=ctrlSharedLib/Kalman Filter  mask(ctrlKalmanFilter){TimeDomain=Discrete-Time, UseCurrentEstimator=off, ModelSource=Input port, ModelSourceVariable=sys, A=0.95*eye(2), B=eye(2), C=eye(2), D=zeros(2), NumberOfStates=15, NumberOfInputs=0, NumberOfOutputs=3, InitialEstimateSource=Input port, X0=0, P0=10, UseK=off, UseGH=off, NumberOfProcessNoiseInputs=2, G=diag([zeros(3,1);ones(12,1)]), TimeInvariantG=off, H=0, TimeInvariantH=on, Q=diag([zeros(3,1);1e-2*ones(3,1);1e-4*ones(3,1);zeros(3,1);1e-5*ones(3,1)]), TimeInvariantQ=off, R=diag([0.001,0.001,0.001]), TimeInvariantR=on, N=0, TimeInvariantN=on, AddInputPort=off, AddEnablePort=on, ExternalReset=Rising, OutputEstimatedY=off, OutputP=on, Ts=dt}
      mask prompts: TimeDomain "Controllib:blocks:maskPromptKFTimeDomain"; UseCurrentEstimator "Controllib:blocks:maskPromptKFUseCurrentMeasurement"; ModelSource "Controllib:blocks:maskPromptKFModelSource"; ModelSourceVariable "Controllib:blocks:maskPromptKFModelSourceVariable"; A "Controllib:blocks:maskPromptKFA"; B "Controllib:blocks:maskPromptKFB"; C "Controllib:blocks:maskPromptKFC"; D "Controllib:blocks:maskPromptKFD"; NumberOfStates "Controllib:blocks:maskPromptKFNumberOfStates"; NumberOfInputs "Controllib:blocks:maskPromptKFNumberOfInputs"; NumberOfOutputs "Controllib:blocks:maskPromptKFNumberOfOutputs"; InitialEstimateSource "Controllib:blocks:maskPromptKFSource"; X0 "Controllib:blocks:maskPromptKFX0DT"; P0 "Controllib:blocks:maskPromptKFP0DT"; UseK "Controllib:blocks:maskPromptKFUseK"; UseGH "Controllib:blocks:maskPromptKFUseGH"; NumberOfProcessNoiseInputs "Controllib:blocks:maskPromptKFNumberOfProcessNoiseInputs"; G "Controllib:blocks:maskPromptKFG"; TimeInvariantG "Controllib:blocks:maskPromptKFTimeInvariantG"; H "Controllib:blocks:maskPromptKFH"; TimeInvariantH "Controllib:blocks:maskPromptKFTimeInvariantH"; Q "Controllib:blocks:maskPromptKFQ"; TimeInvariantQ "Controllib:blocks:maskPromptKFTimeInvariantQ"; R "Controllib:blocks:maskPromptKFR"; TimeInvariantR "Controllib:blocks:maskPromptKFTimeInvariantR"; N "Controllib:blocks:maskPromptKFN"; TimeInvariantN "Controllib:blocks:maskPromptKFTimeInvariantN"; AddInputPort "Controllib:blocks:maskPromptKFAddInputPort"; AddEnablePort "Controllib:blocks:maskPromptKFAddEnablePort"; ExternalReset "Simulink:blkprm_prompts:DelayBlkExternalReset"; OutputEstimatedY "Controllib:blocks:maskPromptKFOutputEstimatedY"; OutputP "Controllib:blocks:maskPromptKFOutputP"; Ts "Controllib:blocks:maskPromptKFTs"
      mask help: Controllib:blocks:maskPromptKFDescription
      mask init:
      | dlgParams.TimeDomain = TimeDomain;
      | dlgParams.UseCurrentEstimator = UseCurrentEstimator;
      | dlgParams.ModelSource = ModelSource;
      | dlgParams.ModelSourceVariable = ModelSourceVariable;
      | dlgParams.A = A;
      | dlgParams.B = B;
      | dlgParams.C = C;
      | dlgParams.D = D;
      | dlgParams.ModelHasFeedthrough = true();
      | dlgParams.NumberOfStates = NumberOfStates;
      | dlgParams.NumberOfInputs = NumberOfInputs;
      | dlgParams.NumberOfOutputs = NumberOfOutputs;
      | dlgParams.InitialEstimateSource = InitialEstimateSource;
      | dlgParams.X0 = X0;
      | dlgParams.P0 = P0;
      | dlgParams.UseGH = UseGH;
      | dlgParams.UseK = UseK;
      | dlgParams.NumberOfProcessNoiseInputs = NumberOfProcessNoiseInputs;
      | dlgParams.G = G;
      | dlgParams.TimeInvariantG = TimeInvariantG;
      | dlgParams.H = H;
      | dlgParams.TimeInvariantH = TimeInvariantH;
      | dlgParams.Q = Q;
      | dlgParams.TimeInvariantQ = TimeInvariantQ;
      | dlgParams.R = R;
      | dlgParams.TimeInvariantR = TimeInvariantR;
      | dlgParams.N = N;
      | dlgParams.TimeInvariantN = TimeInvariantN;
      | % Block options panel
      | dlgParams.OutputEstimatedY = OutputEstimatedY;
      | dlgParams.OutputP = OutputP;
      | dlgParams.AddEnablePort = AddEnablePort;
      | dlgParams.AddInputPort = AddInputPort;
      | dlgParams.ExternalReset = ExternalReset;
      | dlgParams.Ts = Ts;
      | [pInitialization,p] = ...
      |     controllib.internal.blocks.kalmanfilter.maskInitializationFcn(gcbh,dlgParams);
      | % Avoid storing dlg variables twice in the MaskWSVariables 
      | % block property
      | clear dlgParams;
      settings: LibrarySourceBlock=ctrlSharedLib/Kalman Filter
      mask Help: eval('controllib.internal.blocks.kalmanfilter.launchDocPage()')
      mask TypeOptions TimeDomain: Controllib:blocks:maskPromptKFTimeDomainDT | Controllib:blocks:maskPromptKFTimeDomainCT
      mask Callback TimeDomain: controllib.internal.blocks.kalmanfilter.dialogCallbacks(gcbh(),'comboBoxTimeDomain');
      mask Callback UseCurrentEstimator: controllib.internal.blocks.kalmanfilter.dialogCallbacks(gcbh(),'checkBoxUseCurrentEstimator');
      mask TypeOptions ModelSource: Controllib:blocks:maskPromptKFModelSourceLTIObject | Controllib:blocks:maskPromptKFModelSourceMatrices | Controllib:blocks:maskPromptKFSourceInport
      mask Callback ModelSource: controllib.internal.blocks.kalmanfilter.dialogCallbacks(gcbh(),'comboBoxModelSource');
      mask Callback ModelSourceVariable: controllib.internal.blocks.kalmanfilter.dialogCallbacks(gcbh(),'editBoxModelSourceVariable')
      mask TypeOptions InitialEstimateSource: Controllib:blocks:maskPromptKFSourceDialog | Controllib:blocks:maskPromptKFSourceInport
      mask Callback InitialEstimateSource: controllib.internal.blocks.kalmanfilter.dialogCallbacks(gcbh(),'comboBoxInitialEstimateSource');
      mask Callback UseK: controllib.internal.blocks.kalmanfilter.dialogCallbacks(gcbh(),'checkBoxUseK');
      mask Callback UseGH: controllib.internal.blocks.kalmanfilter.dialogCallbacks(gcbh(),'checkBoxUseGH');
      mask Callback TimeInvariantG: controllib.internal.blocks.kalmanfilter.dialogCallbacks(gcbh(),'checkBoxTimeInvariantGH');
      mask Callback TimeInvariantH: controllib.internal.blocks.kalmanfilter.dialogCallbacks(gcbh(),'checkBoxTimeInvariantGH');
      mask Callback TimeInvariantQ: controllib.internal.blocks.kalmanfilter.dialogCallbacks(gcbh(),'checkBoxTimeInvariantQRN');
      mask Callback TimeInvariantR: controllib.internal.blocks.kalmanfilter.dialogCallbacks(gcbh(),'checkBoxTimeInvariantQRN');
      mask Callback TimeInvariantN: controllib.internal.blocks.kalmanfilter.dialogCallbacks(gcbh(),'checkBoxTimeInvariantQRN');
      mask Callback AddInputPort: controllib.internal.blocks.kalmanfilter.dialogCallbacks(gcbh(),'checkBoxAddInputPort');
      mask TypeOptions ExternalReset: MemoryX/ExternalReset
      mask Callback OutputP: controllib.internal.blocks.kalmanfilter.dialogCallbacks(gcbh(),'checkBoxOutputP');
      mask DialogControl DescGroupVar Prompt: Controllib:blocks:maskPromptKFTitle
      mask DialogControl FilterSettingsContainer Prompt: Controllib:blocks:maskPromptKFContainerFilterSettings
      mask DialogControl TimeDomain Prompt: 时域:
      mask DialogControl UseCurrentEstimator Prompt: 使用当前测量 y[n] 来改进 xhat[n]
      mask DialogControl ModelParameterContainer Prompt: Controllib:blocks:maskPromptKFTabModelParameters
      mask DialogControl SystemModelContainer Prompt: Controllib:blocks:maskPromptKFContainerSystemModel
      mask DialogControl ModelSource Prompt: 模型源:
      mask DialogControl ModelSourceVariable Prompt: 变量:
      mask DialogControl A Prompt: A:
      mask DialogControl B Prompt: B:
      mask DialogControl C Prompt: C:
      mask DialogControl D Prompt: D:
      mask DialogControl NumberOfStates Prompt: 状态数量:
      mask DialogControl NumberOfInputs Prompt: 输入数目:
      mask DialogControl NumberOfOutputs Prompt: 输出数目:
      mask DialogControl InitialEstimatesContainer Prompt: Controllib:blocks:maskPromptKFContainerInitialEstimates
      mask DialogControl InitialEstimateSource Prompt: 源:
      mask DialogControl X0 Prompt: 初始状态 x[0]:
      mask DialogControl P0 Prompt: 状态估计误差协方差 P[0]
      mask DialogControl NoiseCharacteristicsContainer Prompt: Controllib:blocks:maskPromptKFContainerNoiseCharacteristics
      mask DialogControl UseK Prompt: 使用来自模型变量的 Kalman 增益 K
      mask DialogControl UseGH Prompt: 使用 G 和 H 矩阵(默认 G=I，H=0)
      mask DialogControl NumberOfProcessNoiseInputs Prompt: 过程噪声输入数目:
      mask DialogControl G Prompt: G:
      mask DialogControl TimeInvariantG Prompt: 时不变 G
      mask DialogControl H Prompt: H:
      mask DialogControl TimeInvariantH Prompt: 时不变 H
      mask DialogControl Q Prompt: Q:
      mask DialogControl TimeInvariantQ Prompt: 时不变 Q
      mask DialogControl R Prompt: R:
      mask DialogControl TimeInvariantR Prompt: 时不变 R
      mask DialogControl N Prompt: N:
      mask DialogControl TimeInvariantN Prompt: 时不变 N
      mask DialogControl OptionsContainer Prompt: Controllib:blocks:maskPromptKFTabOptions
      mask DialogControl AdditionalInportsContainer Prompt: Controllib:blocks:maskPromptKFContainerAdditionalInports
      mask DialogControl AddInputPort Prompt: 添加输入端口 u
      mask DialogControl AddEnablePort Prompt: 添加输入端口 Enable 以控制测量更新
      mask DialogControl ExternalReset Prompt: 外部重置:
      mask DialogControl AdditionalOutportsContainer Prompt: Controllib:blocks:maskPromptKFContainerAdditionalOutports
      mask DialogControl OutputEstimatedY Prompt: 输出估计的模型输出 y
      mask DialogControl OutputP Prompt: 输出状态估计误差协方差 P
      mask DialogControl Ts Prompt: 采样时间(-1 表示继承):
  Logical Operator : Logic  Commented=on  Operator=OR  AllPortsSameDT=off  OutDataTypeStr=boolean
  MATLAB Function : MATLAB Function  TreatAsAtomicUnit=on
  MATLAB Function2 : MATLAB Function  TreatAsAtomicUnit=on
  Memory : Memory
  Mux : Mux  Inputs=3
  Mux1 : Mux  Inputs=3
  Rate Transition : RateTransition  OutPortSampleTime=dt
  Rate Transition1 : RateTransition
  Rate Transition2 : RateTransition  OutPortSampleTime=dt
  Rate Transition3 : RateTransition  OutPortSampleTime=dt
  Scope{,2..3,5,7,9..10} (7 alike) : Scope
  Subsystem : Subsystem
  Terminator : Terminator
  delta_state : Outport
  Measuemrnt Enable Flag : Outport  Port=2
  covariance : Outport  Port=3
  wires:
  Data Store Read2/1 -> Logical Operator/1, GNSS/INS Kalman Filter1/5(Reset)
  Bus Selector/9 -> [QGC_init]  "<QGC_sensor_reinit>"
  Mux/1 -> [pos_NED]
  Rate Transition3/1 -> GNSS/INS Kalman Filter1/4(Enable)
  [Enable] -> Rate Transition3/1
  Memory/1 -> MATLAB Function/1(u)
  Bus Creator/1 -> delta_state/1
  MATLAB Function/3(dtheta) -> Bus Creator/3  "KFState_dtheta"
  Data Type Conversion1/1 -> Memory/1
  MATLAB Function/1(dp) -> Bus Creator/1  "KFState_dp"
  MATLAB Function/5(dg) -> Bus Creator/5  "KFState_da"
  MATLAB Function/2(dv) -> Bus Creator/2  "KFState_dv"
  MATLAB Function/4(da) -> Bus Creator/4  "KFState_da"
  Bus Selector2/3 -> [p_INS]  "<INSstste_p>"
  Bus Selector2/1 -> [DCM_b_n]  "<DCM_b_n>"
  Bus Selector2/5 -> [fbxyz]  "<INSstate_fb>"
  Bus Selector2/4 -> [wxyz]  "<INSstate_w>"
  INS state/1 -> Bus Selector2/1
  [Enable] -> Measuemrnt Enable Flag/1
  Bus Selector/4 -> Mux/3  "<pos_D_gps>"
  Bus Selector/2 -> Mux/1  "<pos_N_gps>"
  Bus Selector/3 -> Mux/2  "<pos_E_gps>"
  Bus Selector/7 -> Mux1/3  "<vd_gps>"
  Bus Selector/5 -> Mux1/1  "<vn_gps>"
  Mux1/1 -> Scope2/1, Terminator/1
  Sensor_data/1 -> Bus Selector/1
  Bus Selector/6 -> Mux1/2  "<ve_gps>"
  Extract Diagonal/1 -> Scope9/1, covariance/1
  GNSS/INS Kalman Filter1/2(P) -> Extract Diagonal/1
  Data Store Read1/1 -> Scope7/1
  Rate Transition2/1 -> Data Type Conversion5/1
  Cal Q/1(Qd) -> Rate Transition2/1
  MATLAB Function2/1(P) -> Data Type Conversion2/1
  Data Type Conversion5/1 -> GNSS/INS Kalman Filter1/8(Q)
  Cal Phi/1(Phi) -> Rate Transition1/1
  [DCM_b_n] -> Cal Phi/1(<DCM_b_n>)
  [pos_NED] -> Subsystem/1(data)
  [fbxyz] -> Cal Phi/3(axyz)
  Data Type Conversion2/1 -> GNSS/INS Kalman Filter1/3(P0)
  [pos_NED] -> Add/2, Scope3/1
  [p_INS] -> Add/1
  Rate Transition1/1 -> Data Type Conversion3/1
  [DCM_b_n] -> Cal Q/1(<DCM_b_n>)
  [wxyz] -> Cal Phi/2(wxyz)
  Add/1 -> Rate Transition/1, Scope10/1
  Data Type Conversion3/1 -> GNSS/INS Kalman Filter1/6(A)
  Constant6/1 -> GNSS/INS Kalman Filter1/7(C)
  [wxyz] -> Cal Q/2(wxyz)
  Rate Transition/1 -> GNSS/INS Kalman Filter1/1(y)
  Subsystem/1(flag) -> [Enable], Scope5/1
  GNSS/INS Kalman Filter1/1(xhat) -> Data Type Conversion1/1, Scope/1
  Constant7/1 -> GNSS/INS Kalman Filter1/2(X0)
